simulink model "test_bench_sponge"  (Simulink 9.2)
settings: Solver=FixedStepDiscrete  StartTime=0.0  StopTime=inf  FixedStep=t_sample_s/10  RelTol=1e-3
values from neighbouring files (symbols this model uses):
  p_max_bar = 0.5    [init.m]
  p_supply_bar = 0.3    [init.m]
  t_sample_s = 1e-3    (= 0.001)    [init.m]
undefined symbols (not defined in the file or in its folder): slave_i2c
libraries: test_bench_lib x25, etherlab_lib x11, pePwmGenerator x7, simulink x6, dspfdesign x5, dspsigops x3
settings Model: Creator=moritz  LastModifiedBy=entwicklungs-pc  SimulationMode=external  ExtModeTrigDuration=100000  ExtModeArchiveMode=auto  ExtModeArchiveFileName=measurement_data  ExtModeArchiveDirName=./results  ExtModeLogAll=off
settings DataIOCC: LimitDataPoints=off  SaveFormat=Dataset  SignalLoggingSaveFormat=Dataset  SaveOutput=off  SignalLogging=off  SaveTime=off
settings OptimizationCC: BlockReduction=off  ConditionallyExecuteInputs=off  OptimizeBlockIOStorage=off  BufferReuse=off  GlobalBufferReuse=off  ExpressionFolding=off  LocalBlockOutputs=off  LifeSpan=auto  OptimizeDataStoreBuffers=off  BusAssignmentInplaceUpdate=off
settings DebuggingCC: UnderspecifiedInitializationDetection=Simplified  MergeDetectMultiDrivingBlocksExec=error  FcnCallInpInsideContextMsg=error  StateNameClashWarn=none  SFUnexpectedBacktrackingDiag=error  SFNoUnconditionalDefaultTransitionDiag=error  SFExecutionAtInitializationDiag=warning
settings HardwareCC: ProdBitPerPointer=64  ProdBitPerSizeT=64  ProdBitPerPtrDiffT=64  ProdLargestAtomicFloat=Float  ProdIntDivRoundTo=Zero  ProdEndianess=LittleEndian  ProdWordSize=64  ProdHWDeviceType=Intel->x86-64 (Windows64)
settings ModelReferenceCC: PropagateSignalLabelsOutOfModel=on
settings RTWCC: SystemTargetFile=etherlab.tlc  TemplateMakefile=etherlab_hrt.tmf  Description=EtherLab PREEMT_RT Real-Time Target
settings CodeAppCC: StateflowObjectComments=off
settings STFCustomTargetCC: TargetLangStandard=C99 (ISO)  ModelReferenceCompliant=off  SystemTargetFile=etherlab.tlc
settings GRTTargetCC: TargetLangStandard=C99 (ISO)  ModelReferenceCompliant=off  ParMdlRefBuildCompliant=off  CompOptLevelCompliant=off  ConcurrentExecutionCompliant=off  GeneratePreprocessorConditionals=Use local settings  MatFileLogging=off  CPPClassGenCompliant=off  UseToolchainInfoCompliant=off  ExtMode=on  ExtModeStaticAlloc=on  ExtModeStaticAllocSize=10000000  ExtModeMexArgs='130.75.144.164' 0 17725  RTWCAPISignals=on  RTWCAPIParams=on
settings CustomProperty: DataType=int32  Value=2
settings ConfigComp: CovMetricSettings=dwe  CovHtmlReporting=off  CovSaveCumulativeToWorkspaceVar=off  CovSaveSingleToWorkspaceVar=off  CovExternalEMLEnable=on

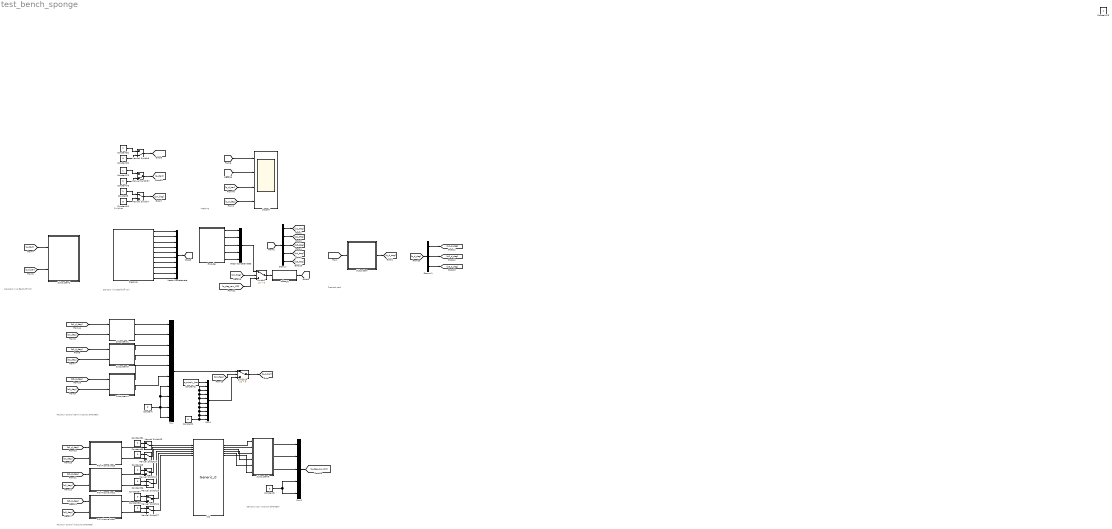
== system test_bench_sponge ==
  note: Sensors (via Beckhoff I/O)
  note: Actuators (via Beckhoff I/O)
  note: Switches
  note: Desired path
  note: Position control (semi-modular SPONGE)
  note: Logging
  note: Position control (modular SPONGE)
  note: Sensors (I2C, modular SPONGE)
  Constant{,1,3,10,20,76} (6 alike) : Constant  Value=0  SampleTime=t_sample_s
  Constant2 : Constant  Value=p_supply_bar  SampleTime=t_sample_s
  Constant31 : Constant  SampleTime=t_sample_s
  Constant{43,54..58} (6 alike) : Constant  Value=0  SampleTime=1e-3
  Constant5 : Constant  SampleTime=t_sample_s
  Constant75 : Constant  SampleTime=t_sample_s
  Constant78 : Constant
  Demux : Demux  Outputs=5
  Demux1 : Demux  Outputs=3
  "Encoder " : Subsystem
  I2C : etherlab_lib/EtherCAT/Generic_0  master=0  index=12  rv=slave_i2c()  param=[]  tsample=t_sample_s  debug=0
  Manual Switch{7,15,23..27} (7 alike) : ManualSwitch
  Manual Switch37 : ManualSwitch  CurrentSetting=0
  Manual Switch8 : ManualSwitch  CurrentSetting=0
  Mux : Mux  Inputs=10
  Mux1 : Mux  Inputs=10
  Mux2 : Mux  Inputs=5
  PID Microvalves1 : Subsystem
  PID Microvalves2 : Subsystem
  PID Microvalves3 : Subsystem
  "Pressure " : Subsystem
  Scope7 : Scope  NumInputPorts=4
  Subsystem : Subsystem
  Subsystem1 : Subsystem
  Subsystem2 : Subsystem
  Subsystem3 : Subsystem
  Subsystem4 : Subsystem
  Subsystem5 : Subsystem
  Switch1 : Switch  Criteria=u2 > Threshold
  Switch14 : Switch  Criteria=u2 > Threshold
  Vector Concatenate : Concatenate  NumInputs=10
  Vector Concatenate3 : Concatenate  NumInputs=5
  offset_q : MATLAB Function  TreatAsAtomicUnit=on
  wires:
  "Pressure "/3("p21_bar ") -> Vector Concatenate/3
  "Pressure "/4(p22_bar) -> Vector Concatenate/4
  "Pressure "/1("p11_bar ") -> Vector Concatenate/1
  "Pressure "/2(p12_bar) -> Vector Concatenate/2
  "Pressure "/5(p31_bar) -> Vector Concatenate/5
  "Pressure "/6(p32_bar) -> Vector Concatenate/6
  "Pressure "/7(p41_bar) -> Vector Concatenate/7
  "Pressure "/8(p42_bar) -> Vector Concatenate/8
  "Pressure "/9(p51_bar) -> Vector Concatenate/9
  "Pressure "/10(p52_bar) -> Vector Concatenate/10
  [p_d_bar] -> Scope7/3  "p_d_bar"
  Constant76/1 -> Manual Switch37/2
  Constant75/1 -> Manual Switch37/1
  Manual Switch37/1 -> [p_start]
  Vector Concatenate/1 -> [p_bar]
  "Encoder "/1(q1_deg_raw) -> Vector Concatenate3/1
  "Encoder "/2(q2_deg_raw) -> Vector Concatenate3/2
  "Encoder "/3(q3_deg_raw) -> Vector Concatenate3/3
  "Encoder "/4(q4_deg_raw) -> Vector Concatenate3/4
  "Encoder "/5(q5_deg_raw) -> Vector Concatenate3/5
  Vector Concatenate3/1 -> Switch1/1  "q_deg_raw"
  offset_q/1(q_deg) -> [q_deg]
  [p_start] -> Subsystem2/1(p_start)
  [p_d_bar] -> Subsystem2/2(p_d_bar)
  [p_bar] -> Scope7/1  "p_bar"
  [q_deg] -> Scope7/2  "q_deg"
  Constant10/1 -> Manual Switch7/2  "m"
  Constant5/1 -> Manual Switch7/1  "sm"
  Manual Switch7/1 -> [sm_flag]
  Manual Switch8/1 -> [global_start]
  Constant31/1 -> Manual Switch8/1
  Constant20/1 -> Manual Switch8/2
  [global_start] -> Subsystem/1(global_start)
  Subsystem/1("q_d_deg ") -> [q_d_deg]
  [q_d_deg] -> Scope7/4  "q_d_deg"
  [q_deg] -> Demux/1
  Demux/1 -> [q1_deg]
  Demux/2 -> [q2_deg]
  Demux/3 -> [q3_deg]
  Demux/4 -> [q4_deg]
  Demux/5 -> [q5_deg]
  [q1_d_deg] -> Subsystem1/1(qi_d_deg)
  [q1_deg] -> Subsystem1/2(qi_deg)
  Subsystem1/1(pi1_d_bar) -> Mux/1  "p11_d_bar"
  Subsystem1/2(pi2_d_bar) -> Mux/2  "p12_d_bar"
  Subsystem3/2(pi2_d_bar) -> Mux/4  "p22_d_bar"
  Subsystem3/1(pi1_d_bar) -> Mux/3  "p21_d_bar"
  [q2_deg] -> Subsystem3/2(qi_deg)
  [q2_d_deg] -> Subsystem3/1(qi_d_deg)
  [q3_d_deg] -> Subsystem4/1(qi_d_deg)
  [q3_deg] -> Subsystem4/2(qi_deg)
  Subsystem4/1(pi1_d_bar) -> Mux/5  "p31_d_bar"
  Subsystem4/2(pi2_d_bar) -> Mux/6  "p32_d_bar"
  Constant/1 -> Mux/10, Mux/7, Mux/8, Mux/9
  Manual Switch24/1 -> I2C/2
  Constant57/1 -> Manual Switch26/1
  PID Microvalves1/1(PWMi1) -> Manual Switch15/2
  PID Microvalves2/1(PWMi1) -> Manual Switch26/2
  Manual Switch27/1 -> I2C/6
  Manual Switch25/1 -> I2C/4
  Manual Switch15/1 -> I2C/3
  PID Microvalves3/2(PWMi2) -> Manual Switch24/2  "PWM2"
  Manual Switch23/1 -> I2C/1
  Manual Switch26/1 -> I2C/5
  Constant58/1 -> Manual Switch27/1
  PID Microvalves2/2(PWMi2) -> Manual Switch27/2
  Constant56/1 -> Manual Switch25/1
  Constant43/1 -> Manual Switch15/1
  PID Microvalves1/2(PWMi2) -> Manual Switch25/2
  [q1_deg] -> PID Microvalves3/2(qi_deg)  "theta_hall_deg"
  PID Microvalves3/1(PWMi1) -> Manual Switch23/2  "PWM1"
  Constant54/1 -> Manual Switch23/1
  Constant55/1 -> Manual Switch24/1
  [q1_d_deg] -> PID Microvalves3/1(qi_d_deg)
  [q2_d_deg] -> PID Microvalves1/1(qi_d_deg)
  [q2_deg] -> PID Microvalves1/2(qi_deg)  "theta_hall_deg"
  [q3_deg] -> PID Microvalves2/2(qi_deg)  "theta_hall_deg"
  [q3_d_deg] -> PID Microvalves2/1(qi_d_deg)
  Mux/1 -> Switch14/1
  Mux1/1 -> Switch14/3
  [sm_flag] -> Switch14/2
  Switch14/1 -> [p_d_bar]
  Constant1/1 -> Mux1/8, Mux1/4, Mux1/2, Mux1/3, Mux1/5, Mux1/6, Mux1/7, Mux1/9, Mux1/10
  Constant2/1 -> Mux1/1
  Switch1/1 -> offset_q/1(q_deg_raw)
  [sm_flag] -> Switch1/2
  [q_deg_raw_I2C] -> Switch1/3
  I2C/1 -> Subsystem5/1("l1 ")  "lowerbyte"
  I2C/2 -> Subsystem5/2(h1)  "upperbyte"
  I2C/3 -> Subsystem5/3(l2)
  I2C/4 -> Subsystem5/4(h2)
  I2C/5 -> Subsystem5/5("l3 ")
  I2C/6 -> Subsystem5/6("h3 ")
  Subsystem5/1(Out1) -> Mux2/1
  Subsystem5/2(Out2) -> Mux2/2
  Subsystem5/3(Out3) -> Mux2/3
  Constant3/1 -> Mux2/4, Mux2/5
  Mux2/1 -> [q_deg_raw_I2C]
  [q_d_deg] -> Demux1/1
  Demux1/1 -> [q1_d_deg]
  Demux1/2 -> [q2_d_deg]
  Demux1/3 -> [q3_d_deg]

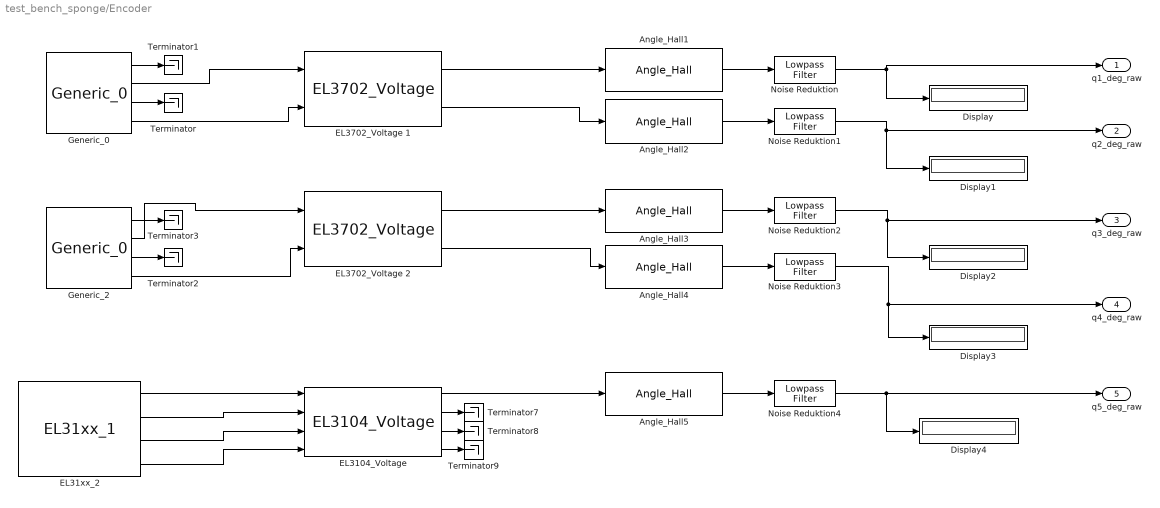
== system test_bench_sponge/Encoder  ==
  Angle_Hall{1..5} (5 alike) : test_bench_lib/Angle_Hall  SystemSampleTime=-1
  Display{,1..4} (5 alike) : Display
  EL3104_Voltage : test_bench_lib/EL3104_Voltage  SystemSampleTime=-1
  EL31xx_2 : etherlab_lib/EtherCAT/Beckhoff/EL31xx_1  master=0  index=8  model=EL3104  revision=[203436114 1179648]  vector=off  status=off  filter=Off  gain=[]  offset=[]  tau=[]  tsample=t_sample_s  debug=0  dc_mode=Free Run/SM-Synchron  dc_assign_activate=hex2dec('700')  dc_cycle0=[]  dc_cycle0_factor=[]  dc_shift0=[]  dc_shift0_factor=[]  dc_shift0_input=off  dc_cycle1=[]  dc_cycle1_factor=[]  dc_shift1=[]  dc_shift1_factor=[]
      settings: AttributesFormatString=|
      | EL3104
      | M:0 Idx:8
  EL3702_Voltage 1 : test_bench_lib/EL3702_Voltage  SystemSampleTime=-1
  EL3702_Voltage 2 : test_bench_lib/EL3702_Voltage  SystemSampleTime=-1
  Generic_0 : etherlab_lib/EtherCAT/Generic_0  master=0  index=6  rv=slave_el3102  param=[]  tsample=t_sample_s  debug=0
  Generic_2 : etherlab_lib/EtherCAT/Generic_0  master=0  index=7  rv=slave_el3102  param=[]  tsample=t_sample_s  debug=0
  Noise Reduktion{,1..4} (5 alike) : dspfdesign/Lowpass Filter  FilterType=FIR  DesignForMinimumOrder=on  FilterOrder=50  PassbandFrequency=0.1  StopbandFrequency=5  PassbandRipple=0.1  StopbandAttenuation=60  InheritSampleRate=off  SampleRate=1000  SimulateUsing=Interpreted execution  roundingMode=Floor  coeffsDataTypeStr=fixdt(1,16)
  Terminator{,1..3,7..9} (7 alike) : Terminator
  q1_deg_raw : Outport
  q2_deg_raw : Outport  Port=2
  q3_deg_raw : Outport  Port=3
  q4_deg_raw : Outport  Port=4
  q5_deg_raw : Outport  Port=5
  wires:
  EL3702_Voltage 1/1 -> Angle_Hall1/1
  Angle_Hall1/1 -> Noise Reduktion/1
  Noise Reduktion/1 -> q1_deg_raw/1, Display/1
  Noise Reduktion3/1 -> q4_deg_raw/1, Display3/1
  Generic_0/4 -> EL3702_Voltage 1/2
  EL3702_Voltage 2/1 -> Angle_Hall3/1
  Generic_2/4 -> EL3702_Voltage 2/2
  Noise Reduktion1/1 -> Display1/1, q2_deg_raw/1
  Angle_Hall3/1 -> Noise Reduktion2/1
  EL31xx_2/1 -> EL3104_Voltage/1
  Noise Reduktion4/1 -> q5_deg_raw/1, Display4/1
  EL3104_Voltage/3 -> Terminator8/1
  Angle_Hall4/1 -> Noise Reduktion3/1
  Generic_0/3 -> Terminator/1
  Generic_0/2 -> EL3702_Voltage 1/1
  EL3702_Voltage 1/2 -> Angle_Hall2/1
  Angle_Hall5/1 -> Noise Reduktion4/1
  Generic_2/3 -> Terminator2/1
  Noise Reduktion2/1 -> q3_deg_raw/1, Display2/1
  EL3104_Voltage/2 -> Terminator7/1
  EL3104_Voltage/1 -> Angle_Hall5/1
  EL3702_Voltage 2/2 -> Angle_Hall4/1
  Generic_2/1 -> Terminator3/1
  Generic_0/1 -> Terminator1/1
  Angle_Hall2/1 -> Noise Reduktion1/1
  Generic_2/2 -> EL3702_Voltage 2/1
  EL3104_Voltage/4 -> Terminator9/1
  EL31xx_2/2 -> EL3104_Voltage/2
  EL31xx_2/3 -> EL3104_Voltage/3
  EL31xx_2/4 -> EL3104_Voltage/4

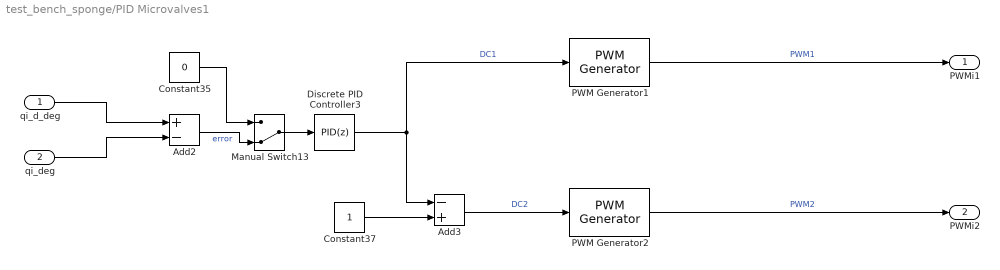
== system test_bench_sponge/PID Microvalves1 ==
  qi_d_deg : Inport
  qi_deg : Inport  Port=2
  Add2 : Sum  Inputs=+-
  Add3 : Sum  Inputs=-+
  Constant35 : Constant  Value=0
  Constant37 : Constant
  Discrete PID Controller3 : simulink/Continuous/PID Controller  Controller=PID  Form=Parallel  TimeDomain=Discrete-time  SampleTime=-1  IntegratorMethod=Forward Euler  FilterMethod=Forward Euler  ControllerParametersSource=internal  P=3e-2  I=3e-2  D=0  UseFilter=on  N=100  TunerSelectOption=Transfer Function Based (PID Tuner App)  InitialConditionSource=internal  InitialConditionForIntegrator=0  InitialConditionForFilter=0  DifferentiatorICPrevScaledInput=0  ExternalReset=none  TrackingMode=off  Kt=1  LimitOutput=on  UpperSaturationLimit=1  LowerSaturationLimit=0  LinearizeAsGain=off  AntiWindupMode=back-calculation  Kb=1  POutMin=[]  POutMax=[]  IOutMin=[]  IOutMax=[]  DOutMin=[]  DOutMax=[]  NOutMin=[]  NOutMax=[]  SumOutMin=[]  SumOutMax=[]  SaturationOutMin=[]  SaturationOutMax=[]  PParamMin=[]  PParamMax=[]  IParamMin=[]  IParamMax=[]  DParamMin=[]  DParamMax=[]  NParamMin=[]  NParamMax=[]  KbParamMin=[]  KbParamMax=[]  KtParamMin=[]  KtParamMax=[]  KbOutMin=[]  KbOutMax=[]  KtOutMin=[]  KtOutMax=[]  IntegratorOutMin=[]  IntegratorOutMax=[]  FilterOutMin=[]  FilterOutMax=[]  SumI1OutMin=[]  SumI1OutMax=[]  SumI2OutMin=[]  SumI2OutMax=[]  SumI3OutMin=[]  SumI3OutMax=[]  SumI4OutMin=[]  SumI4OutMax=[]  SumDOutMin=[]  SumDOutMax=[]  DifferentiatorOutMin=[]  DifferentiatorOutMax=[]  FilterDiffOutCoefMin=[]  FilterDiffOutCoefMax=[]  ReciprocalOutMin=[]  ReciprocalOutMax=[]  SumDenOutMin=[]  SumDenOutMax=[]  SumNumOutMin=[]  SumNumOutMax=[]  DivideOutMin=[]  DivideOutMax=[]  IntegratorContinuousStateAttributes=''  IntegratorStateMustResolveToSignalObject=off  IntegratorRTWStateStorageClass=Auto  FilterContinuousStateAttributes=''  FilterStateMustResolveToSignalObject=off  FilterRTWStateStorageClass=Auto  ParallelPVariant=InternalParameters  IdealPVariant=Disabled  IVariant=InternalParameters  DVariant=InternalParameters  IntegratorVariant=Discrete  SatVariant=Enabled  AWVariant=BackCalculation  PCopyVariant=Disabled  TRVariant=Disabled  FdbkBlocksVariant=Forward  IdealPFdbkVariant=Disabled  SatFdbkVariant=Disabled  DerivativeFilterVariant=ForwardEulerFilter  NVariant=InternalParameters  NCopyVariant=Disabled  FilterICVariant=InternalICsFilter  IntegratorICVariant=InternalICs  ExternalResetVariant=Disabled  TRSumVariant=Passthrough  SumFdbkVariant=Disabled  SumVariant=Sum_PID
  Manual Switch13 : ManualSwitch  CurrentSetting=0
  PWM Generator1 : pePwmGenerator/PWM Generator  CarrCount=Up  Tper=t_PWM_s  Ts=t_sample_s/10
  PWM Generator2 : pePwmGenerator/PWM Generator  CarrCount=Up  Tper=t_PWM_s  Ts=t_sample_s/10
  PWMi1 : Outport
  PWMi2 : Outport  Port=2
  wires:
  Constant35/1 -> Manual Switch13/1
  Add2/1 -> Manual Switch13/2  "error"
  Discrete PID Controller3/1 -> PWM Generator1/1, Add3/1  "DC1"
  Manual Switch13/1 -> Discrete PID Controller3/1
  qi_d_deg/1 -> Add2/1
  qi_deg/1 -> Add2/2
  Constant37/1 -> Add3/2
  Add3/1 -> PWM Generator2/1  "DC2"
  PWM Generator1/1 -> PWMi1/1  "PWM1"
  PWM Generator2/1 -> PWMi2/1  "PWM2"

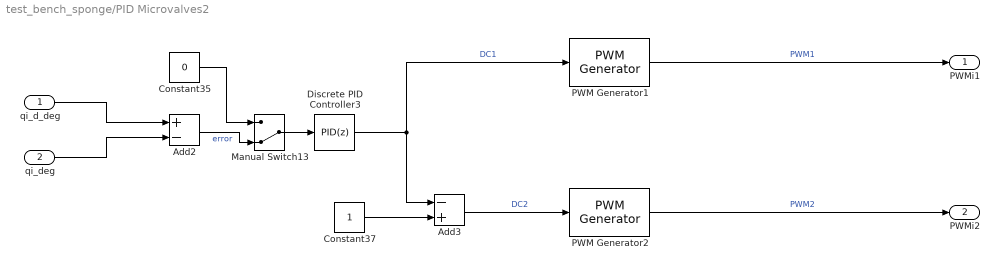
== system test_bench_sponge/PID Microvalves2 ==
  qi_d_deg : Inport
  qi_deg : Inport  Port=2
  Add2 : Sum  Inputs=+-
  Add3 : Sum  Inputs=-+
  Constant35 : Constant  Value=0
  Constant37 : Constant
  Discrete PID Controller3 : simulink/Continuous/PID Controller  Controller=PID  Form=Parallel  TimeDomain=Discrete-time  SampleTime=-1  IntegratorMethod=Forward Euler  FilterMethod=Forward Euler  ControllerParametersSource=internal  P=3e-2  I=3e-2  D=0  UseFilter=on  N=100  TunerSelectOption=Transfer Function Based (PID Tuner App)  InitialConditionSource=internal  InitialConditionForIntegrator=0  InitialConditionForFilter=0  DifferentiatorICPrevScaledInput=0  ExternalReset=none  TrackingMode=off  Kt=1  LimitOutput=on  UpperSaturationLimit=1  LowerSaturationLimit=0  LinearizeAsGain=off  AntiWindupMode=back-calculation  Kb=1  POutMin=[]  POutMax=[]  IOutMin=[]  IOutMax=[]  DOutMin=[]  DOutMax=[]  NOutMin=[]  NOutMax=[]  SumOutMin=[]  SumOutMax=[]  SaturationOutMin=[]  SaturationOutMax=[]  PParamMin=[]  PParamMax=[]  IParamMin=[]  IParamMax=[]  DParamMin=[]  DParamMax=[]  NParamMin=[]  NParamMax=[]  KbParamMin=[]  KbParamMax=[]  KtParamMin=[]  KtParamMax=[]  KbOutMin=[]  KbOutMax=[]  KtOutMin=[]  KtOutMax=[]  IntegratorOutMin=[]  IntegratorOutMax=[]  FilterOutMin=[]  FilterOutMax=[]  SumI1OutMin=[]  SumI1OutMax=[]  SumI2OutMin=[]  SumI2OutMax=[]  SumI3OutMin=[]  SumI3OutMax=[]  SumI4OutMin=[]  SumI4OutMax=[]  SumDOutMin=[]  SumDOutMax=[]  DifferentiatorOutMin=[]  DifferentiatorOutMax=[]  FilterDiffOutCoefMin=[]  FilterDiffOutCoefMax=[]  ReciprocalOutMin=[]  ReciprocalOutMax=[]  SumDenOutMin=[]  SumDenOutMax=[]  SumNumOutMin=[]  SumNumOutMax=[]  DivideOutMin=[]  DivideOutMax=[]  IntegratorContinuousStateAttributes=''  IntegratorStateMustResolveToSignalObject=off  IntegratorRTWStateStorageClass=Auto  FilterContinuousStateAttributes=''  FilterStateMustResolveToSignalObject=off  FilterRTWStateStorageClass=Auto  ParallelPVariant=InternalParameters  IdealPVariant=Disabled  IVariant=InternalParameters  DVariant=InternalParameters  IntegratorVariant=Discrete  SatVariant=Enabled  AWVariant=BackCalculation  PCopyVariant=Disabled  TRVariant=Disabled  FdbkBlocksVariant=Forward  IdealPFdbkVariant=Disabled  SatFdbkVariant=Disabled  DerivativeFilterVariant=ForwardEulerFilter  NVariant=InternalParameters  NCopyVariant=Disabled  FilterICVariant=InternalICsFilter  IntegratorICVariant=InternalICs  ExternalResetVariant=Disabled  TRSumVariant=Passthrough  SumFdbkVariant=Disabled  SumVariant=Sum_PID
  Manual Switch13 : ManualSwitch  CurrentSetting=0
  PWM Generator1 : pePwmGenerator/PWM Generator  CarrCount=Up  Tper=t_PWM_s  Ts=t_sample_s/10
  PWM Generator2 : pePwmGenerator/PWM Generator  CarrCount=Up  Tper=t_PWM_s  Ts=t_sample_s/10
  PWMi1 : Outport
  PWMi2 : Outport  Port=2
  wires:
  PWM Generator2/1 -> PWMi2/1  "PWM2"
  PWM Generator1/1 -> PWMi1/1  "PWM1"
  Add3/1 -> PWM Generator2/1  "DC2"
  Constant37/1 -> Add3/2
  qi_deg/1 -> Add2/2
  qi_d_deg/1 -> Add2/1
  Manual Switch13/1 -> Discrete PID Controller3/1
  Discrete PID Controller3/1 -> PWM Generator1/1, Add3/1  "DC1"
  Add2/1 -> Manual Switch13/2  "error"
  Constant35/1 -> Manual Switch13/1

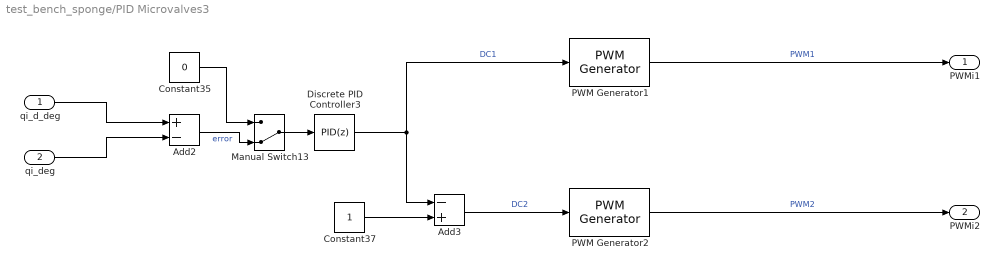
== system test_bench_sponge/PID Microvalves3 ==
  qi_d_deg : Inport
  qi_deg : Inport  Port=2
  Add2 : Sum  Inputs=+-
  Add3 : Sum  Inputs=-+
  Constant35 : Constant  Value=0
  Constant37 : Constant
  Discrete PID Controller3 : simulink/Continuous/PID Controller  Controller=PID  Form=Parallel  TimeDomain=Discrete-time  SampleTime=-1  IntegratorMethod=Forward Euler  FilterMethod=Forward Euler  ControllerParametersSource=internal  P=2e-2  I=3e-2  D=0  UseFilter=on  N=100  TunerSelectOption=Transfer Function Based (PID Tuner App)  InitialConditionSource=internal  InitialConditionForIntegrator=0  InitialConditionForFilter=0  DifferentiatorICPrevScaledInput=0  ExternalReset=none  TrackingMode=off  Kt=1  LimitOutput=on  UpperSaturationLimit=1  LowerSaturationLimit=0  LinearizeAsGain=off  AntiWindupMode=back-calculation  Kb=1  POutMin=[]  POutMax=[]  IOutMin=[]  IOutMax=[]  DOutMin=[]  DOutMax=[]  NOutMin=[]  NOutMax=[]  SumOutMin=[]  SumOutMax=[]  SaturationOutMin=[]  SaturationOutMax=[]  PParamMin=[]  PParamMax=[]  IParamMin=[]  IParamMax=[]  DParamMin=[]  DParamMax=[]  NParamMin=[]  NParamMax=[]  KbParamMin=[]  KbParamMax=[]  KtParamMin=[]  KtParamMax=[]  KbOutMin=[]  KbOutMax=[]  KtOutMin=[]  KtOutMax=[]  IntegratorOutMin=[]  IntegratorOutMax=[]  FilterOutMin=[]  FilterOutMax=[]  SumI1OutMin=[]  SumI1OutMax=[]  SumI2OutMin=[]  SumI2OutMax=[]  SumI3OutMin=[]  SumI3OutMax=[]  SumI4OutMin=[]  SumI4OutMax=[]  SumDOutMin=[]  SumDOutMax=[]  DifferentiatorOutMin=[]  DifferentiatorOutMax=[]  FilterDiffOutCoefMin=[]  FilterDiffOutCoefMax=[]  ReciprocalOutMin=[]  ReciprocalOutMax=[]  SumDenOutMin=[]  SumDenOutMax=[]  SumNumOutMin=[]  SumNumOutMax=[]  DivideOutMin=[]  DivideOutMax=[]  IntegratorContinuousStateAttributes=''  IntegratorStateMustResolveToSignalObject=off  IntegratorRTWStateStorageClass=Auto  FilterContinuousStateAttributes=''  FilterStateMustResolveToSignalObject=off  FilterRTWStateStorageClass=Auto  ParallelPVariant=InternalParameters  IdealPVariant=Disabled  IVariant=InternalParameters  DVariant=InternalParameters  IntegratorVariant=Discrete  SatVariant=Enabled  AWVariant=BackCalculation  PCopyVariant=Disabled  TRVariant=Disabled  FdbkBlocksVariant=Forward  IdealPFdbkVariant=Disabled  SatFdbkVariant=Disabled  DerivativeFilterVariant=ForwardEulerFilter  NVariant=InternalParameters  NCopyVariant=Disabled  FilterICVariant=InternalICsFilter  IntegratorICVariant=InternalICs  ExternalResetVariant=Disabled  TRSumVariant=Passthrough  SumFdbkVariant=Disabled  SumVariant=Sum_PID
  Manual Switch13 : ManualSwitch  CurrentSetting=0
  PWM Generator1 : pePwmGenerator/PWM Generator  CarrCount=Up  Tper=t_PWM_s  Ts=t_sample_s/10
  PWM Generator2 : pePwmGenerator/PWM Generator  CarrCount=Up  Tper=t_PWM_s  Ts=t_sample_s/10
  PWMi1 : Outport
  PWMi2 : Outport  Port=2
  wires:
  PWM Generator2/1 -> PWMi2/1  "PWM2"
  PWM Generator1/1 -> PWMi1/1  "PWM1"
  Add3/1 -> PWM Generator2/1  "DC2"
  Constant37/1 -> Add3/2
  qi_deg/1 -> Add2/2
  qi_d_deg/1 -> Add2/1
  Manual Switch13/1 -> Discrete PID Controller3/1
  Discrete PID Controller3/1 -> PWM Generator1/1, Add3/1  "DC1"
  Add2/1 -> Manual Switch13/2  "error"
  Constant35/1 -> Manual Switch13/1

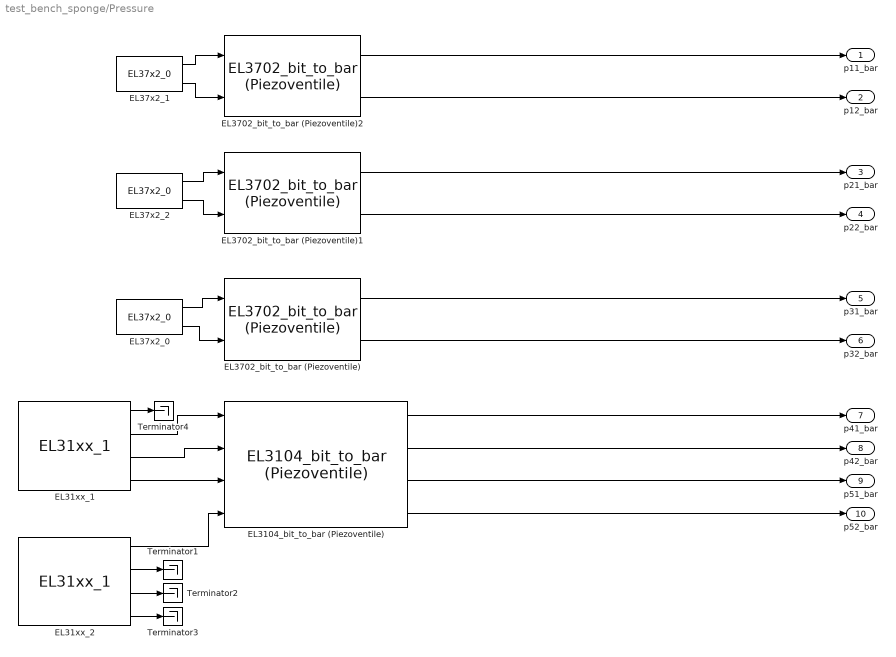
== system test_bench_sponge/Pressure  ==
  EL3104_bit_to_bar (Piezoventile) : test_bench_lib/EL3104_bit_to_bar (Piezoventile)  SystemSampleTime=-1
  EL31xx_1 : etherlab_lib/EtherCAT/Beckhoff/EL31xx_1  master=0  index=8  model=EL3104  revision=[203436114 1179648]  vector=off  status=off  filter=Off  gain=[]  offset=[]  tau=[]  tsample=t_sample_s  debug=0  dc_mode=Free Run/SM-Synchron  dc_assign_activate=hex2dec('700')  dc_cycle0=[]  dc_cycle0_factor=[]  dc_shift0=[]  dc_shift0_factor=[]  dc_shift0_input=off  dc_cycle1=[]  dc_cycle1_factor=[]  dc_shift1=[]  dc_shift1_factor=[]
      settings: AttributesFormatString=|
      | EL3104
      | M:0 Idx:8
  EL31xx_2 : etherlab_lib/EtherCAT/Beckhoff/EL31xx_1  master=0  index=9  model=EL3104  revision=[203436114 1179648]  vector=off  status=off  filter=Off  gain=[]  offset=[]  tau=[]  tsample=t_sample_s  debug=0  dc_mode=Free Run/SM-Synchron  dc_assign_activate=hex2dec('700')  dc_cycle0=[]  dc_cycle0_factor=[]  dc_shift0=[]  dc_shift0_factor=[]  dc_shift0_input=off  dc_cycle1=[]  dc_cycle1_factor=[]  dc_shift1=[]  dc_shift1_factor=[]
      settings: AttributesFormatString=|
      | EL3104
      | M:0 Idx:9
  EL3702_bit_to_bar (Piezoventile) : test_bench_lib/EL3702_bit_to_bar (Piezoventile)  SystemSampleTime=-1
  EL3702_bit_to_bar (Piezoventile)1 : test_bench_lib/EL3702_bit_to_bar (Piezoventile)  SystemSampleTime=-1
  EL3702_bit_to_bar (Piezoventile)2 : test_bench_lib/EL3702_bit_to_bar (Piezoventile)  SystemSampleTime=-1
  EL37x2_0 : etherlab_lib/EtherCAT/Beckhoff/EL37x2_0  master=0  index=5  model=EL3702  revision=[242626642 131072]  one_ch=off  scale=[]  offset=[]  tsample=t_sample_s  debug=0  dc_mode=1  dc_assign_activate=hex2dec('730')  dc_cycle0=0  dc_cycle0_factor="-10     % 10-times OS"  dc_shift0=-10000  dc_shift0_factor=1  dc_shift0_input=off  dc_cycle1=0  dc_cycle1_factor=-1  dc_shift1=0  dc_shift1_factor=0
  EL37x2_1 : etherlab_lib/EtherCAT/Beckhoff/EL37x2_0  master=0  index=3  model=EL3702  revision=[242626642 131072]  one_ch=off  scale=[]  offset=[]  tsample=t_sample_s  debug=0  dc_mode=1  dc_assign_activate=hex2dec('730')  dc_cycle0=0  dc_cycle0_factor="-10     % 10-times OS"  dc_shift0=-10000  dc_shift0_factor=1  dc_shift0_input=off  dc_cycle1=0  dc_cycle1_factor=-1  dc_shift1=0  dc_shift1_factor=0
  EL37x2_2 : etherlab_lib/EtherCAT/Beckhoff/EL37x2_0  master=0  index=4  model=EL3702  revision=[242626642 131072]  one_ch=off  scale=[]  offset=[]  tsample=t_sample_s  debug=0  dc_mode=1  dc_assign_activate=hex2dec('730')  dc_cycle0=0  dc_cycle0_factor="-10     % 10-times OS"  dc_shift0=-10000  dc_shift0_factor=1  dc_shift0_input=off  dc_cycle1=0  dc_cycle1_factor=-1  dc_shift1=0  dc_shift1_factor=0
  Terminator{1..4} (4 alike) : Terminator
  "p11_bar " : Outport
  p12_bar : Outport  Port=2
  "p21_bar " : Outport  Port=3
  p22_bar : Outport  Port=4
  p31_bar : Outport  Port=5
  p32_bar : Outport  Port=6
  p41_bar : Outport  Port=7
  p42_bar : Outport  Port=8
  p51_bar : Outport  Port=9
  p52_bar : Outport  Port=10
  wires:
  EL37x2_0/1 -> EL3702_bit_to_bar (Piezoventile)/1
  EL3702_bit_to_bar (Piezoventile)/2 -> p32_bar/1
  EL3702_bit_to_bar (Piezoventile)/1 -> p31_bar/1
  EL37x2_0/2 -> EL3702_bit_to_bar (Piezoventile)/2
  EL37x2_1/2 -> EL3702_bit_to_bar (Piezoventile)2/2
  EL37x2_1/1 -> EL3702_bit_to_bar (Piezoventile)2/1
  EL3702_bit_to_bar (Piezoventile)1/2 -> p22_bar/1
  EL37x2_2/2 -> EL3702_bit_to_bar (Piezoventile)1/2
  EL37x2_2/1 -> EL3702_bit_to_bar (Piezoventile)1/1
  EL3702_bit_to_bar (Piezoventile)1/1 -> "p21_bar "/1
  EL3702_bit_to_bar (Piezoventile)2/1 -> "p11_bar "/1
  EL3702_bit_to_bar (Piezoventile)2/2 -> p12_bar/1
  EL3104_bit_to_bar (Piezoventile)/2 -> p42_bar/1
  EL3104_bit_to_bar (Piezoventile)/1 -> p41_bar/1
  EL3104_bit_to_bar (Piezoventile)/4 -> p52_bar/1
  EL3104_bit_to_bar (Piezoventile)/3 -> p51_bar/1
  EL31xx_1/2 -> EL3104_bit_to_bar (Piezoventile)/1
  EL31xx_1/3 -> EL3104_bit_to_bar (Piezoventile)/2
  EL31xx_1/4 -> EL3104_bit_to_bar (Piezoventile)/3
  EL31xx_2/1 -> EL3104_bit_to_bar (Piezoventile)/4
  EL31xx_2/2 -> Terminator1/1
  EL31xx_2/3 -> Terminator2/1
  EL31xx_2/4 -> Terminator3/1
  EL31xx_1/1 -> Terminator4/1

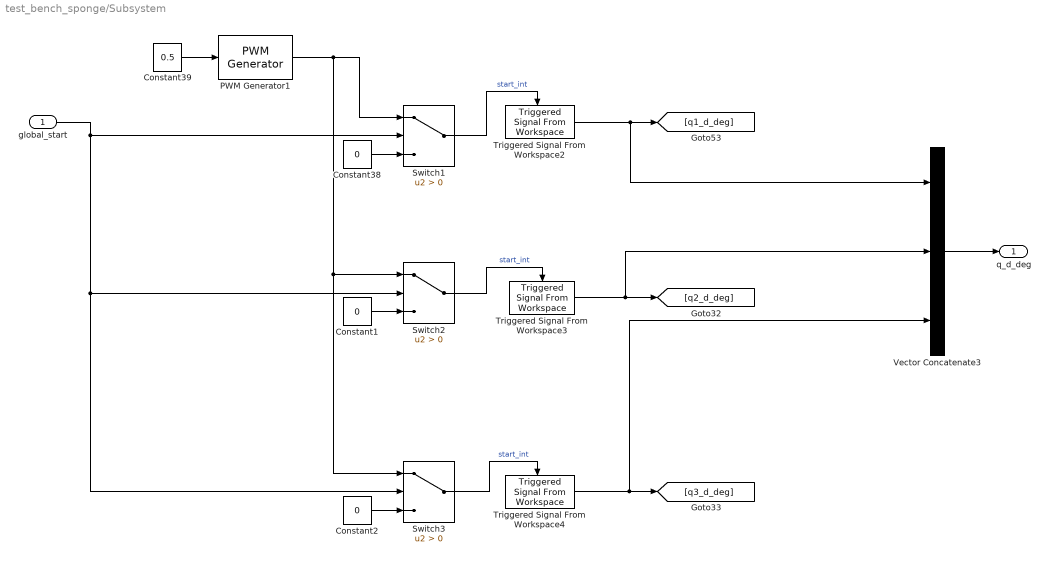
== system test_bench_sponge/Subsystem ==
  global_start : Inport
  Constant1 : Constant  Value=0  SampleTime=1e-3
  Constant2 : Constant  Value=0  SampleTime=1e-3
  Constant38 : Constant  Value=0  SampleTime=1e-3
  Constant39 : Constant  Value=0.5  SampleTime=1e-4
  PWM Generator1 : pePwmGenerator/PWM Generator  CarrCount=Up  Tper=0.05  Ts=t_sample_s/10
  Switch1 : Switch  Criteria=u2 > Threshold
  Switch2 : Switch  Criteria=u2 > Threshold
  Switch3 : Switch  Criteria=u2 > Threshold
  Triggered Signal From Workspace2 : dspsigops/Triggered Signal From Workspace  Signal=q1_d_deg_all  TriggerType=Rising edge  ic=0  SamplesPerFrame=1  OutputAfterFinalValue=Cyclic repetition  OutputFrames=off
      settings: SourceProductName=DSP System Toolbox  SourceProductBaseCode=DS
  Triggered Signal From Workspace3 : dspsigops/Triggered Signal From Workspace  Signal=q2_d_deg_all  TriggerType=Rising edge  ic=0  SamplesPerFrame=1  OutputAfterFinalValue=Cyclic repetition  OutputFrames=off
      settings: SourceProductName=DSP System Toolbox  SourceProductBaseCode=DS
  Triggered Signal From Workspace4 : dspsigops/Triggered Signal From Workspace  Signal=q3_d_deg_all  TriggerType=Rising edge  ic=0  SamplesPerFrame=1  OutputAfterFinalValue=Cyclic repetition  OutputFrames=off
      settings: SourceProductName=DSP System Toolbox  SourceProductBaseCode=DS
  Vector Concatenate3 : Concatenate  NumInputs=3
  "q_d_deg " : Outport
  wires:
  Constant2/1 -> Switch3/3
  Constant39/1 -> PWM Generator1/1
  Triggered Signal From Workspace2/1 -> Vector Concatenate3/1, [q1_d_deg]
  PWM Generator1/1 -> Switch3/1, Switch2/1, Switch1/1
  Triggered Signal From Workspace4/1 -> Vector Concatenate3/3, [q3_d_deg]
  Constant1/1 -> Switch2/3
  Switch1/1 -> Triggered Signal From Workspace2/Trigger  "start_int"
  global_start/1 -> Switch3/2, Switch2/2, Switch1/2
  Switch2/1 -> Triggered Signal From Workspace3/Trigger  "start_int"
  Triggered Signal From Workspace3/1 -> Vector Concatenate3/2, [q2_d_deg]
  Constant38/1 -> Switch1/3
  Switch3/1 -> Triggered Signal From Workspace4/Trigger  "start_int"
  Vector Concatenate3/1 -> "q_d_deg "/1

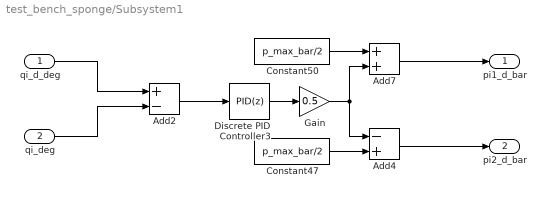
== system test_bench_sponge/Subsystem1 ==
  qi_d_deg : Inport
  qi_deg : Inport  Port=2
  Add2 : Sum  Inputs=+-
  Add4 : Sum  Inputs=-+
  Add7 : Sum
  Constant47 : Constant  Value=p_max_bar/2
  Constant50 : Constant  Value=p_max_bar/2
  Discrete PID Controller3 : simulink/Continuous/PID Controller  Controller=PID  Form=Parallel  TimeDomain=Discrete-time  SampleTime=-1  IntegratorMethod=Forward Euler  FilterMethod=Forward Euler  ControllerParametersSource=internal  P=4e-2  I=3e-2  D=0  UseFilter=on  N=100  TunerSelectOption=Transfer Function Based (PID Tuner App)  InitialConditionSource=internal  InitialConditionForIntegrator=0  InitialConditionForFilter=0  DifferentiatorICPrevScaledInput=0  ExternalReset=none  TrackingMode=off  Kt=1  LimitOutput=on  UpperSaturationLimit=p_max_bar  LowerSaturationLimit=-p_max_bar  LinearizeAsGain=off  AntiWindupMode=back-calculation  Kb=1  POutMin=[]  POutMax=[]  IOutMin=[]  IOutMax=[]  DOutMin=[]  DOutMax=[]  NOutMin=[]  NOutMax=[]  SumOutMin=[]  SumOutMax=[]  SaturationOutMin=[]  SaturationOutMax=[]  PParamMin=[]  PParamMax=[]  IParamMin=[]  IParamMax=[]  DParamMin=[]  DParamMax=[]  NParamMin=[]  NParamMax=[]  KbParamMin=[]  KbParamMax=[]  KtParamMin=[]  KtParamMax=[]  KbOutMin=[]  KbOutMax=[]  KtOutMin=[]  KtOutMax=[]  IntegratorOutMin=[]  IntegratorOutMax=[]  FilterOutMin=[]  FilterOutMax=[]  SumI1OutMin=[]  SumI1OutMax=[]  SumI2OutMin=[]  SumI2OutMax=[]  SumI3OutMin=[]  SumI3OutMax=[]  SumI4OutMin=[]  SumI4OutMax=[]  SumDOutMin=[]  SumDOutMax=[]  DifferentiatorOutMin=[]  DifferentiatorOutMax=[]  FilterDiffOutCoefMin=[]  FilterDiffOutCoefMax=[]  ReciprocalOutMin=[]  ReciprocalOutMax=[]  SumDenOutMin=[]  SumDenOutMax=[]  SumNumOutMin=[]  SumNumOutMax=[]  DivideOutMin=[]  DivideOutMax=[]  IntegratorContinuousStateAttributes=''  IntegratorStateMustResolveToSignalObject=off  IntegratorRTWStateStorageClass=Auto  FilterContinuousStateAttributes=''  FilterStateMustResolveToSignalObject=off  FilterRTWStateStorageClass=Auto  ParallelPVariant=InternalParameters  IdealPVariant=Disabled  IVariant=InternalParameters  DVariant=InternalParameters  IntegratorVariant=Discrete  SatVariant=Enabled  AWVariant=BackCalculation  PCopyVariant=Disabled  TRVariant=Disabled  FdbkBlocksVariant=Forward  IdealPFdbkVariant=Disabled  SatFdbkVariant=Disabled  DerivativeFilterVariant=ForwardEulerFilter  NVariant=InternalParameters  NCopyVariant=Disabled  FilterICVariant=InternalICsFilter  IntegratorICVariant=InternalICs  ExternalResetVariant=Disabled  TRSumVariant=Passthrough  SumFdbkVariant=Disabled  SumVariant=Sum_PID
  Gain : Gain  Gain=0.5
  pi1_d_bar : Outport
  pi2_d_bar : Outport  Port=2
  wires:
  qi_d_deg/1 -> Add2/1
  qi_deg/1 -> Add2/2
  Constant50/1 -> Add7/1
  Constant47/1 -> Add4/2
  Gain/1 -> Add7/2, Add4/1
  Discrete PID Controller3/1 -> Gain/1
  Add7/1 -> pi1_d_bar/1
  Add2/1 -> Discrete PID Controller3/1
  Add4/1 -> pi2_d_bar/1

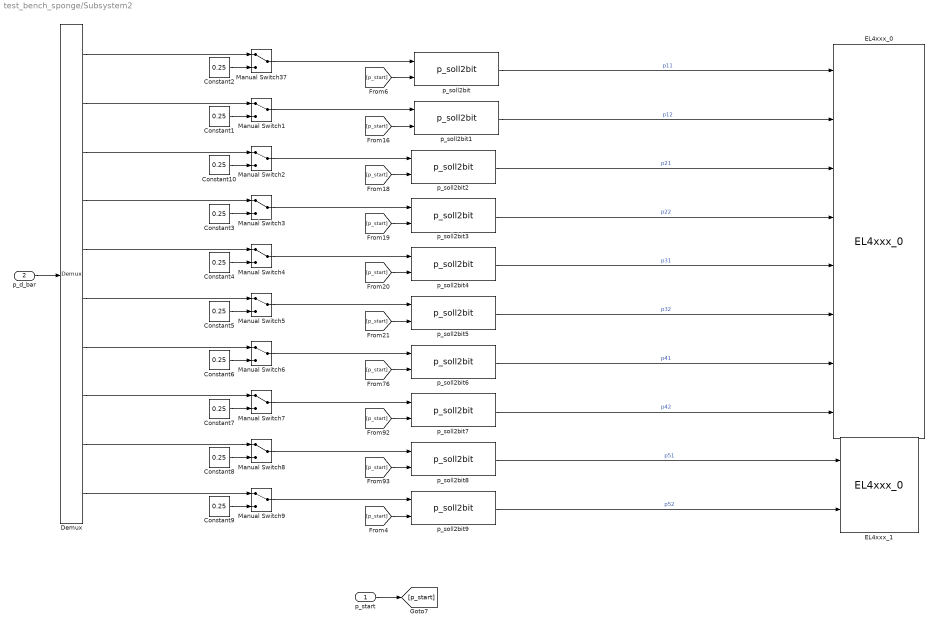
== system test_bench_sponge/Subsystem2 ==
  p_start : Inport
  p_d_bar : Inport  Port=2
  Constant{1..10} (10 alike) : Constant  Value=0.25
  Demux : Demux  Outputs=10
  EL4xxx_0 : etherlab_lib/EtherCAT/Beckhoff/EL4xxx_0  master=0  index=10  model=EL4008  revision=[262680658 1245184]  vector=off  scale=[]  tsample=t_sample_s  debug=0  dc_mode=Free Run  dc_assign_activate=hex2dec('700')  dc_cycle0=0  dc_cycle0_factor=1  dc_shift0=0  dc_shift0_factor=0  dc_shift0_input=off  dc_cycle1=0  dc_cycle1_factor=1  dc_shift1=10000  dc_shift1_factor=0
  EL4xxx_1 : etherlab_lib/EtherCAT/Beckhoff/EL4xxx_0  master=0  index=11  model=EL4102  revision=[268841042 66715648]  vector=off  scale=[]  tsample=t_sample_s  debug=0  dc_mode=Free Run  dc_assign_activate=hex2dec('700')  dc_cycle0=0  dc_cycle0_factor=1  dc_shift0=0  dc_shift0_factor=0  dc_shift0_input=off  dc_cycle1=0  dc_cycle1_factor=1  dc_shift1=10000  dc_shift1_factor=0
  Manual Switch{1..9,37} (10 alike) : ManualSwitch
  p_soll2bit{,1..9} (10 alike) : test_bench_lib/p_soll2bit  SystemSampleTime=-1
  wires:
  [p_start] -> p_soll2bit3/2
  p_soll2bit9/1 -> EL4xxx_1/2  "p52"
  p_soll2bit7/1 -> EL4xxx_0/8  "p42"
  p_soll2bit5/1 -> EL4xxx_0/6  "p32"
  [p_start] -> p_soll2bit9/2
  [p_start] -> p_soll2bit6/2
  p_soll2bit6/1 -> EL4xxx_0/7  "p41"
  [p_start] -> p_soll2bit8/2
  p_soll2bit8/1 -> EL4xxx_1/1  "p51"
  [p_start] -> p_soll2bit2/2
  p_soll2bit4/1 -> EL4xxx_0/5  "p31"
  p_soll2bit3/1 -> EL4xxx_0/4  "p22"
  Demux/4 -> Manual Switch3/1
  [p_start] -> p_soll2bit1/2
  p_soll2bit/1 -> EL4xxx_0/1  "p11"
  Demux/5 -> Manual Switch4/1
  p_soll2bit1/1 -> EL4xxx_0/2  "p12"
  p_soll2bit2/1 -> EL4xxx_0/3  "p21"
  [p_start] -> p_soll2bit7/2
  Demux/1 -> Manual Switch37/1
  p_start/1 -> [p_start]
  [p_start] -> p_soll2bit4/2
  Demux/9 -> Manual Switch8/1
  [p_start] -> p_soll2bit5/2
  [p_start] -> p_soll2bit/2
  Demux/8 -> Manual Switch7/1
  Demux/7 -> Manual Switch6/1
  Demux/2 -> Manual Switch1/1
  Demux/10 -> Manual Switch9/1
  Demux/6 -> Manual Switch5/1
  Demux/3 -> Manual Switch2/1
  p_d_bar/1 -> Demux/1
  Manual Switch37/1 -> p_soll2bit/1
  Manual Switch1/1 -> p_soll2bit1/1
  Manual Switch2/1 -> p_soll2bit2/1
  Manual Switch3/1 -> p_soll2bit3/1
  Manual Switch4/1 -> p_soll2bit4/1
  Manual Switch5/1 -> p_soll2bit5/1
  Manual Switch6/1 -> p_soll2bit6/1
  Manual Switch7/1 -> p_soll2bit7/1
  Manual Switch8/1 -> p_soll2bit8/1
  Constant2/1 -> Manual Switch37/2
  Constant1/1 -> Manual Switch1/2
  Constant10/1 -> Manual Switch2/2
  Constant3/1 -> Manual Switch3/2
  Constant4/1 -> Manual Switch4/2
  Constant5/1 -> Manual Switch5/2
  Constant6/1 -> Manual Switch6/2
  Constant7/1 -> Manual Switch7/2
  Constant8/1 -> Manual Switch8/2
  Constant9/1 -> Manual Switch9/2
  Manual Switch9/1 -> p_soll2bit9/1

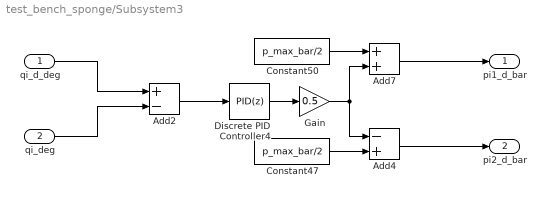
== system test_bench_sponge/Subsystem3 ==
  qi_d_deg : Inport
  qi_deg : Inport  Port=2
  Add2 : Sum  Inputs=+-
  Add4 : Sum  Inputs=-+
  Add7 : Sum
  Constant47 : Constant  Value=p_max_bar/2
  Constant50 : Constant  Value=p_max_bar/2
  Discrete PID Controller4 : simulink/Continuous/PID Controller  Controller=PID  Form=Parallel  TimeDomain=Discrete-time  SampleTime=-1  IntegratorMethod=Forward Euler  FilterMethod=Forward Euler  ControllerParametersSource=internal  P=4e-2  I=2e-2  D=0  UseFilter=on  N=100  TunerSelectOption=Transfer Function Based (PID Tuner App)  InitialConditionSource=internal  InitialConditionForIntegrator=0  InitialConditionForFilter=0  DifferentiatorICPrevScaledInput=0  ExternalReset=none  TrackingMode=off  Kt=1  LimitOutput=on  UpperSaturationLimit=p_max_bar  LowerSaturationLimit=-p_max_bar  LinearizeAsGain=off  AntiWindupMode=back-calculation  Kb=1  POutMin=[]  POutMax=[]  IOutMin=[]  IOutMax=[]  DOutMin=[]  DOutMax=[]  NOutMin=[]  NOutMax=[]  SumOutMin=[]  SumOutMax=[]  SaturationOutMin=[]  SaturationOutMax=[]  PParamMin=[]  PParamMax=[]  IParamMin=[]  IParamMax=[]  DParamMin=[]  DParamMax=[]  NParamMin=[]  NParamMax=[]  KbParamMin=[]  KbParamMax=[]  KtParamMin=[]  KtParamMax=[]  KbOutMin=[]  KbOutMax=[]  KtOutMin=[]  KtOutMax=[]  IntegratorOutMin=[]  IntegratorOutMax=[]  FilterOutMin=[]  FilterOutMax=[]  SumI1OutMin=[]  SumI1OutMax=[]  SumI2OutMin=[]  SumI2OutMax=[]  SumI3OutMin=[]  SumI3OutMax=[]  SumI4OutMin=[]  SumI4OutMax=[]  SumDOutMin=[]  SumDOutMax=[]  DifferentiatorOutMin=[]  DifferentiatorOutMax=[]  FilterDiffOutCoefMin=[]  FilterDiffOutCoefMax=[]  ReciprocalOutMin=[]  ReciprocalOutMax=[]  SumDenOutMin=[]  SumDenOutMax=[]  SumNumOutMin=[]  SumNumOutMax=[]  DivideOutMin=[]  DivideOutMax=[]  IntegratorContinuousStateAttributes=''  IntegratorStateMustResolveToSignalObject=off  IntegratorRTWStateStorageClass=Auto  FilterContinuousStateAttributes=''  FilterStateMustResolveToSignalObject=off  FilterRTWStateStorageClass=Auto  ParallelPVariant=InternalParameters  IdealPVariant=Disabled  IVariant=InternalParameters  DVariant=InternalParameters  IntegratorVariant=Discrete  SatVariant=Enabled  AWVariant=BackCalculation  PCopyVariant=Disabled  TRVariant=Disabled  FdbkBlocksVariant=Forward  IdealPFdbkVariant=Disabled  SatFdbkVariant=Disabled  DerivativeFilterVariant=ForwardEulerFilter  NVariant=InternalParameters  NCopyVariant=Disabled  FilterICVariant=InternalICsFilter  IntegratorICVariant=InternalICs  ExternalResetVariant=Disabled  TRSumVariant=Passthrough  SumFdbkVariant=Disabled  SumVariant=Sum_PID
  Gain : Gain  Gain=0.5
  pi1_d_bar : Outport
  pi2_d_bar : Outport  Port=2
  wires:
  Add4/1 -> pi2_d_bar/1
  Add2/1 -> Discrete PID Controller4/1
  Add7/1 -> pi1_d_bar/1
  Discrete PID Controller4/1 -> Gain/1
  Gain/1 -> Add4/1, Add7/2
  Constant47/1 -> Add4/2
  Constant50/1 -> Add7/1
  qi_deg/1 -> Add2/2
  qi_d_deg/1 -> Add2/1

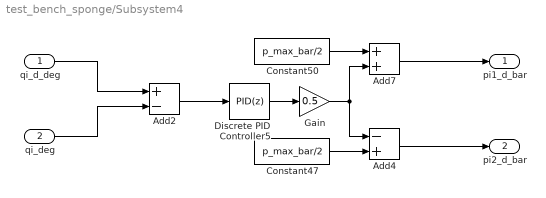
== system test_bench_sponge/Subsystem4 ==
  qi_d_deg : Inport
  qi_deg : Inport  Port=2
  Add2 : Sum  Inputs=+-
  Add4 : Sum  Inputs=-+
  Add7 : Sum
  Constant47 : Constant  Value=p_max_bar/2
  Constant50 : Constant  Value=p_max_bar/2
  Discrete PID Controller5 : simulink/Continuous/PID Controller  Controller=PID  Form=Parallel  TimeDomain=Discrete-time  SampleTime=-1  IntegratorMethod=Forward Euler  FilterMethod=Forward Euler  ControllerParametersSource=internal  P=4e-2  I=3e-2  D=0  UseFilter=on  N=100  TunerSelectOption=Transfer Function Based (PID Tuner App)  InitialConditionSource=internal  InitialConditionForIntegrator=0  InitialConditionForFilter=0  DifferentiatorICPrevScaledInput=0  ExternalReset=none  TrackingMode=off  Kt=1  LimitOutput=on  UpperSaturationLimit=p_max_bar  LowerSaturationLimit=-p_max_bar  LinearizeAsGain=off  AntiWindupMode=back-calculation  Kb=1  POutMin=[]  POutMax=[]  IOutMin=[]  IOutMax=[]  DOutMin=[]  DOutMax=[]  NOutMin=[]  NOutMax=[]  SumOutMin=[]  SumOutMax=[]  SaturationOutMin=[]  SaturationOutMax=[]  PParamMin=[]  PParamMax=[]  IParamMin=[]  IParamMax=[]  DParamMin=[]  DParamMax=[]  NParamMin=[]  NParamMax=[]  KbParamMin=[]  KbParamMax=[]  KtParamMin=[]  KtParamMax=[]  KbOutMin=[]  KbOutMax=[]  KtOutMin=[]  KtOutMax=[]  IntegratorOutMin=[]  IntegratorOutMax=[]  FilterOutMin=[]  FilterOutMax=[]  SumI1OutMin=[]  SumI1OutMax=[]  SumI2OutMin=[]  SumI2OutMax=[]  SumI3OutMin=[]  SumI3OutMax=[]  SumI4OutMin=[]  SumI4OutMax=[]  SumDOutMin=[]  SumDOutMax=[]  DifferentiatorOutMin=[]  DifferentiatorOutMax=[]  FilterDiffOutCoefMin=[]  FilterDiffOutCoefMax=[]  ReciprocalOutMin=[]  ReciprocalOutMax=[]  SumDenOutMin=[]  SumDenOutMax=[]  SumNumOutMin=[]  SumNumOutMax=[]  DivideOutMin=[]  DivideOutMax=[]  IntegratorContinuousStateAttributes=''  IntegratorStateMustResolveToSignalObject=off  IntegratorRTWStateStorageClass=Auto  FilterContinuousStateAttributes=''  FilterStateMustResolveToSignalObject=off  FilterRTWStateStorageClass=Auto  ParallelPVariant=InternalParameters  IdealPVariant=Disabled  IVariant=InternalParameters  DVariant=InternalParameters  IntegratorVariant=Discrete  SatVariant=Enabled  AWVariant=BackCalculation  PCopyVariant=Disabled  TRVariant=Disabled  FdbkBlocksVariant=Forward  IdealPFdbkVariant=Disabled  SatFdbkVariant=Disabled  DerivativeFilterVariant=ForwardEulerFilter  NVariant=InternalParameters  NCopyVariant=Disabled  FilterICVariant=InternalICsFilter  IntegratorICVariant=InternalICs  ExternalResetVariant=Disabled  TRSumVariant=Passthrough  SumFdbkVariant=Disabled  SumVariant=Sum_PID
  Gain : Gain  Gain=0.5
  pi1_d_bar : Outport
  pi2_d_bar : Outport  Port=2
  wires:
  qi_d_deg/1 -> Add2/1
  qi_deg/1 -> Add2/2
  Constant50/1 -> Add7/1
  Constant47/1 -> Add4/2
  Gain/1 -> Add7/2, Add4/1
  Discrete PID Controller5/1 -> Gain/1
  Add7/1 -> pi1_d_bar/1
  Add2/1 -> Discrete PID Controller5/1
  Add4/1 -> pi2_d_bar/1

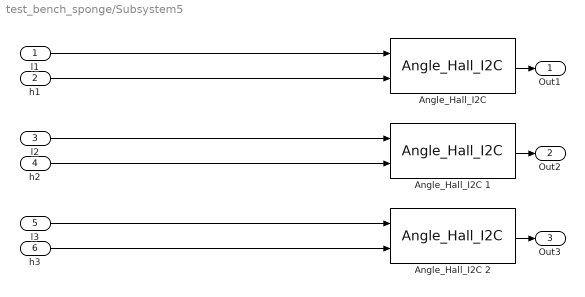
== system test_bench_sponge/Subsystem5 ==
  "l1 " : Inport
  h1 : Inport  Port=2
  l2 : Inport  Port=3
  h2 : Inport  Port=4
  "l3 " : Inport  Port=5
  "h3 " : Inport  Port=6
  "Angle_Hall_I2C " : test_bench_lib/Angle_Hall_I2C   SystemSampleTime=-1
  Angle_Hall_I2C 1 : test_bench_lib/Angle_Hall_I2C   SystemSampleTime=-1
  Angle_Hall_I2C 2 : test_bench_lib/Angle_Hall_I2C   SystemSampleTime=-1
  Out1 : Outport
  Out2 : Outport  Port=2
  Out3 : Outport  Port=3
  wires:
  "l3 "/1 -> Angle_Hall_I2C 2/1
  h2/1 -> Angle_Hall_I2C 1/2
  Angle_Hall_I2C 2/1 -> Out3/1
  "Angle_Hall_I2C "/1 -> Out1/1
  "h3 "/1 -> Angle_Hall_I2C 2/2
  l2/1 -> Angle_Hall_I2C 1/1
  h1/1 -> "Angle_Hall_I2C "/2
  Angle_Hall_I2C 1/1 -> Out2/1
  "l1 "/1 -> "Angle_Hall_I2C "/1

== matlab function offset_q ==
  data: q_deg_raw input double; q_deg output double; offset_q parameter double
function q_deg = subtract_offset(q_deg_raw,offset_q)
q_deg = q_deg_raw-offset_q';
